simulink model "modQPSKspectre"  (Simulink 10.1)
settings: Solver=FixedStepDiscrete  StartTime=0.0  StopTime=inf  RelTol=1e-3
libraries: commutil2 x4, dspsrcs4 x4, commrandsrc3 x2, simulink x2, commfilt2 x2
settings Model: Creator=iba  LastModifiedBy=iba
settings DataIOCC: SaveFormat=Dataset  ReturnWorkspaceOutputs=on
settings OptimizationCC: LifeSpan=auto
settings DebuggingCC: UnderspecifiedInitializationDetection=Simplified  MergeDetectMultiDrivingBlocksExec=error  SFUnexpectedBacktrackingDiag=error  SFNoUnconditionalDefaultTransitionDiag=error  SFExecutionAtInitializationDiag=warning  ArithmeticOperatorsInVariantConditions=error
settings HardwareCC: ProdBitPerPointer=64  ProdBitPerSizeT=64  ProdBitPerPtrDiffT=64  ProdLargestAtomicFloat=Float  ProdIntDivRoundTo=Zero  ProdEndianess=LittleEndian  ProdWordSize=64  ProdHWDeviceType=Intel->x86-64 (Windows64)
settings ModelReferenceCC: PropagateSignalLabelsOutOfModel=on
settings SFSimCC: SimUseLocalCustomCode=on  CustomCodeUndefinedFunction=FilterOut
settings RTWCC: RTWUseLocalCustomCode=on
settings CodeAppCC: StateflowObjectComments=off
settings GRTTargetCC: TargetLangStandard=C99 (ISO)  CombineOutputUpdateFcns=on  GRTInterface=off
settings ConfigComp: CovMetricSettings=dwe  CovHtmlReporting=off  CovSaveCumulativeToWorkspaceVar=off  CovSaveSingleToWorkspaceVar=off  CovExternalEMLEnable=on

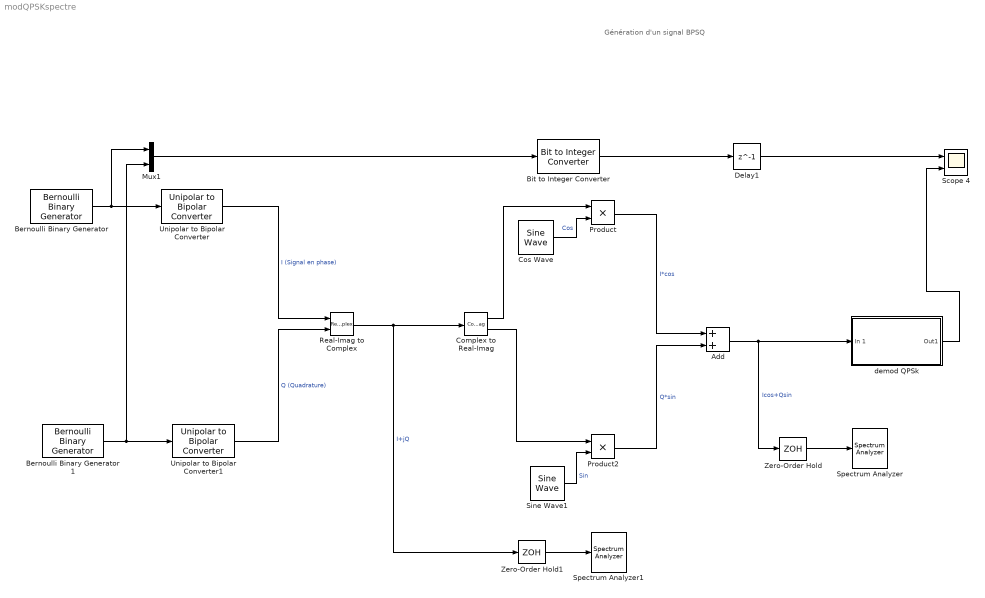
== system modQPSKspectre ==
  note: Génération d'un signal BPSQ
  Add : Sum
  "Bernoulli Binary Generator " : commrandsrc3/Bernoulli Binary Generator  ProbabilityOfZero=0.5  SeedSource=Parameter  Seed=23  SampleTime=1  SamplesPerFrame=1  OutputDataType=double  SimulateUsing=Interpreted execution
  Bernoulli Binary Generator 1 : commrandsrc3/Bernoulli Binary Generator  ProbabilityOfZero=0.5  SeedSource=Parameter  Seed=61  SampleTime=1  SamplesPerFrame=1  OutputDataType=double  SimulateUsing=Interpreted execution
  Bit to Integer Converter : commutil2/Bit to Integer Converter  nbits=2  bitOrder=MSB first  signedOutputValues=Unsigned  outDtype=double  outDtypeSigned=Inherit via internal rule
  Complex to Real-Imag : ComplexToRealImag
  Cos Wave : dspsrcs4/Sine Wave  Amplitude=1  Frequency=5  Phase=pi/2  SampleMode=Discrete  OutComplex=Real  CompMethod=Trigonometric fcn  TableSize=Speed  SampleTime=1/100  SamplesPerFrame=1  ResetState=Restart at time zero  OutputFrames=off  dataType=double  wordLen=16  udDataType=sfix(16)  fracBitsMode=Best precision  numFracBits=15  OutDataTypeStr=double  LastOutDataTypeStr=double
  Delay1 : Delay  DelayLength=1  InitialCondition=0
  Mux1 : Mux  Inputs=2
  Product : Product
  Product2 : Product
  Real-Imag to Complex : RealImagToComplex
  Scope 4 : Scope  NumInputPorts=2
  Sine Wave1 : dspsrcs4/Sine Wave  Amplitude=1  Frequency=5  Phase=0  SampleMode=Discrete  OutComplex=Real  CompMethod=Trigonometric fcn  TableSize=Speed  SampleTime=1/100  SamplesPerFrame=1  ResetState=Restart at time zero  OutputFrames=off  dataType=double  wordLen=16  udDataType=sfix(16)  fracBitsMode=Best precision  numFracBits=15  OutDataTypeStr=double  LastOutDataTypeStr=double
  Spectrum Analyzer : SpectrumAnalyzer
  Spectrum Analyzer1 : SpectrumAnalyzer
  Unipolar to Bipolar Converter : commutil2/Unipolar to Bipolar Converter  M=2  polarity=Positive  dataType=Inherit via internal rule
  Unipolar to Bipolar Converter1 : commutil2/Unipolar to Bipolar Converter  M=2  polarity=Positive  dataType=Inherit via internal rule
  Zero-Order Hold : ZeroOrderHold  SampleTime=1/20
  Zero-Order Hold1 : ZeroOrderHold  SampleTime=1/20
  demod QPSk : Subsystem
  wires:
  Unipolar to Bipolar Converter/1 -> Real-Imag to Complex/1  "I (Signal en phase)"
  Cos Wave/1 -> Product/2  "Cos"
  "Bernoulli Binary Generator "/1 -> Mux1/1, Unipolar to Bipolar Converter/1
  Delay1/1 -> Scope 4/1
  Sine Wave1/1 -> Product2/2  "Sin"
  Unipolar to Bipolar Converter1/1 -> Real-Imag to Complex/2  "Q (Quadrature)"
  Bernoulli Binary Generator 1/1 -> Mux1/2, Unipolar to Bipolar Converter1/1
  Product/1 -> Add/1  "I*cos"
  Product2/1 -> Add/2  "Q*sin"
  Mux1/1 -> Bit to Integer Converter/1
  Bit to Integer Converter/1 -> Delay1/1
  Add/1 -> Zero-Order Hold/1, demod QPSk/1(In 1)  "Icos+Qsin"
  demod QPSk/1("Out1 ") -> Scope 4/2
  Complex to Real-Imag/1 -> Product/1
  Complex to Real-Imag/2 -> Product2/1
  Zero-Order Hold1/1 -> Spectrum Analyzer1/1
  Real-Imag to Complex/1 -> Zero-Order Hold1/1, Complex to Real-Imag/1  "I+jQ"
  Zero-Order Hold/1 -> Spectrum Analyzer/1

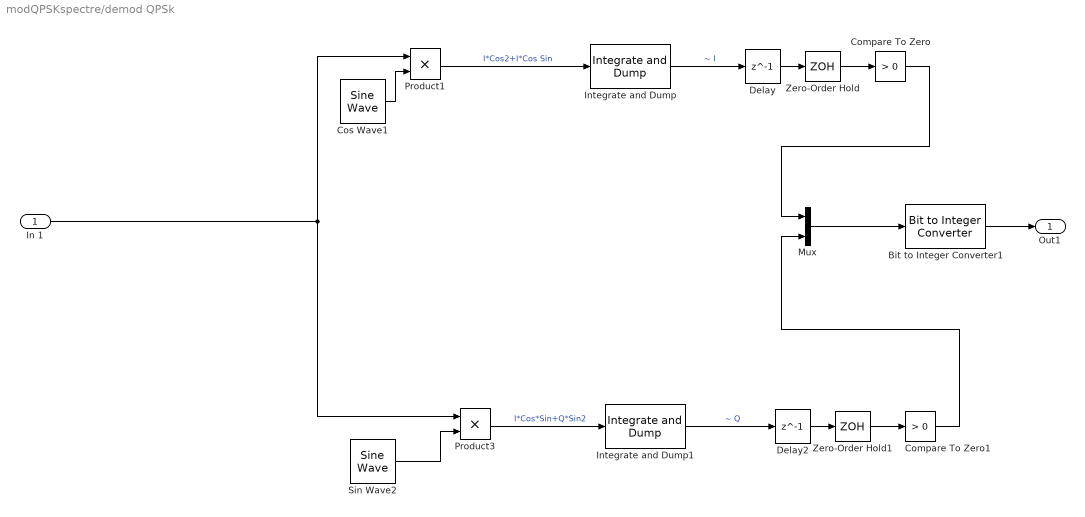
== system modQPSKspectre/demod QPSk ==
  In 1 : Inport
  Bit to Integer Converter1 : commutil2/Bit to Integer Converter  nbits=2  bitOrder=MSB first  signedOutputValues=Unsigned  outDtype=double  outDtypeSigned=Inherit via internal rule
  Compare To Zero : simulink/Logic and Bit Operations/Compare To Zero  relop=>  OutDataTypeStr=boolean
  Compare To Zero1 : simulink/Logic and Bit Operations/Compare To Zero  relop=>  OutDataTypeStr=boolean
  Cos Wave1 : dspsrcs4/Sine Wave  Amplitude=1  Frequency=5  Phase=pi/2  SampleMode=Discrete  OutComplex=Real  CompMethod=Trigonometric fcn  TableSize=Speed  SampleTime=1/100  SamplesPerFrame=1  ResetState=Restart at time zero  OutputFrames=off  dataType=double  wordLen=16  udDataType=sfix(16)  fracBitsMode=Best precision  numFracBits=15  OutDataTypeStr=double  LastOutDataTypeStr=double
  Delay : Delay  DelayLength=1  InitialCondition=0
  Delay2 : Delay  DelayLength=1  InitialCondition=0
  Integrate and Dump : commfilt2/Integrate and Dump  obssamples=100  offsetsamples=0  nodump=on  roundingMode=Floor  overflowMode=off  outputDataTypeStr=Inherit: Same as accumulator  outputLastDataTypeStr=Inherit: Same as accumulator
  Integrate and Dump1 : commfilt2/Integrate and Dump  obssamples=100  offsetsamples=0  nodump=on  roundingMode=Floor  overflowMode=off  outputDataTypeStr=Inherit: Same as accumulator  outputLastDataTypeStr=Inherit: Same as accumulator
  Mux : Mux  Inputs=2
  Product1 : Product
  Product3 : Product
  Sin Wave2 : dspsrcs4/Sine Wave  Amplitude=1  Frequency=5  Phase=0  SampleMode=Discrete  OutComplex=Real  CompMethod=Trigonometric fcn  TableSize=Speed  SampleTime=1/100  SamplesPerFrame=1  ResetState=Restart at time zero  OutputFrames=off  dataType=double  wordLen=16  udDataType=sfix(16)  fracBitsMode=Best precision  numFracBits=15  OutDataTypeStr=double  LastOutDataTypeStr=double
  Zero-Order Hold : ZeroOrderHold
  Zero-Order Hold1 : ZeroOrderHold
  "Out1 " : Outport
  wires:
  Integrate and Dump1/1 -> Delay2/1  "~ Q"
  Zero-Order Hold1/1 -> Compare To Zero1/1
  Sin Wave2/1 -> Product3/2
  Product1/1 -> Integrate and Dump/1  "I*Cos2+I*Cos Sin"
  Delay2/1 -> Zero-Order Hold1/1
  Cos Wave1/1 -> Product1/2
  Product3/1 -> Integrate and Dump1/1  "I*Cos*Sin+Q*Sin2"
  Integrate and Dump/1 -> Delay/1  "~ I"
  Zero-Order Hold/1 -> Compare To Zero/1
  Delay/1 -> Zero-Order Hold/1
  In 1/1 -> Product3/1, Product1/1
  Compare To Zero/1 -> Mux/1
  Mux/1 -> Bit to Integer Converter1/1
  Compare To Zero1/1 -> Mux/2
  Bit to Integer Converter1/1 -> "Out1 "/1
